simulink model "zero_to_hero_sect11_pid"  (R2023a)
settings: Solver=VariableStepAuto  StartTime=0.0  StopTime=simtime  MaxStep=0.01  RelTol=1e-3
values from neighbouring files (symbols this model uses):
  b = 50    [zero_to_hero_sect10_script.m]    (also in zero_to_hero_sect1to5_script.m = 0.1; zero_to_hero_sect7to8_script.m = 10)
undefined symbols (not defined in the file or in its folder): J_Mo, K_m, L, R, target_angular_vel
libraries: slpidlib x1
settings Model: Creator=fycce  LastModifiedBy=fycce
settings DataIOCC: SaveOutput=off  SaveTime=off  ReturnWorkspaceOutputs=off

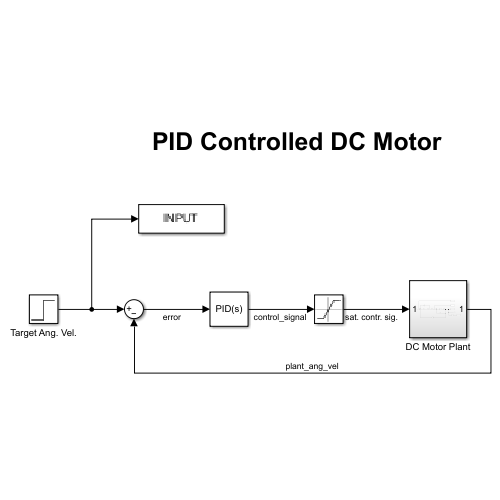
[thumbnail: Simulink's stored preview of the top-level diagram]
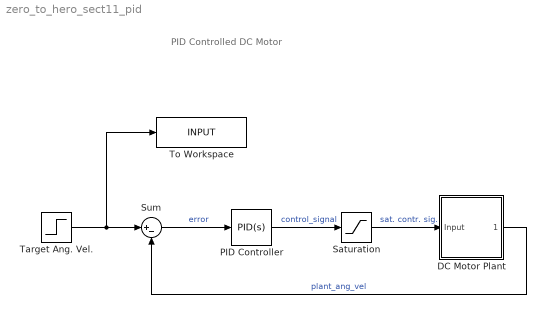
== system zero_to_hero_sect11_pid ==
  note: PID Controlled DC Motor
  DC Motor Plant : Subsystem
  PID Controller : slpidlib/PID Controller  Controller=PID  Form=Parallel  TimeDomain=Continuous-time  UseExternalTs=off  SampleTime=-1  IntegratorMethod=Forward Euler  FilterMethod=Forward Euler  ControllerParametersSource=internal  P=17.19  I=204.8  UseKiTs=off  D=0.2523  N=1422  UseFilter=on  TunerSelectOption=Transfer Function Based (PID Tuner App)  InitialConditionSource=internal  InitialConditionForIntegrator=0  InitialConditionForFilter=0  DifferentiatorICPrevScaledInput=0  ExternalReset=none  TrackingMode=off  Kt=1  LimitOutput=off  SatLimitsSource=internal  UpperSaturationLimit=inf  LowerSaturationLimit=-inf  LinearizeAsGain=on  AntiWindupMode=none  Kb=1  LimitIntegrator=off  UpperIntegratorSaturationLimit=inf  LowerIntegratorSaturationLimit=-inf  POutMin=[]  POutMax=[]  IOutMin=[]  IOutMax=[]  DOutMin=[]  DOutMax=[]  NOutMin=[]  NOutMax=[]  SumOutMin=[]  SumOutMax=[]  SaturationOutMin=[]  SaturationOutMax=[]  PParamMin=[]  PParamMax=[]  IParamMin=[]  IParamMax=[]  DParamMin=[]  DParamMax=[]  NParamMin=[]  NParamMax=[]  KbParamMin=[]  KbParamMax=[]  KtParamMin=[]  KtParamMax=[]  KbOutMin=[]  KbOutMax=[]  KtOutMin=[]  KtOutMax=[]  IntegratorOutMin=[]  IntegratorOutMax=[]  FilterOutMin=[]  FilterOutMax=[]  SumI1OutMin=[]  SumI1OutMax=[]  SumI2OutMin=[]  SumI2OutMax=[]  SumI3OutMin=[]  SumI3OutMax=[]  SumI4OutMin=[]  SumI4OutMax=[]  SumDOutMin=[]  SumDOutMax=[]  DifferentiatorOutMin=[]  DifferentiatorOutMax=[]  FilterDiffOutCoefMin=[]  FilterDiffOutCoefMax=[]  ReciprocalOutMin=[]  ReciprocalOutMax=[]  SumDenOutMin=[]  SumDenOutMax=[]  SumNumOutMin=[]  SumNumOutMax=[]  DivideOutMin=[]  DivideOutMax=[]  UdiffTsProdOutMin=[]  UdiffTsProdOutMax=[]  NTsProdOutMin=[]  NTsProdOutMax=[]  UintegralTsProdOutMin=[]  UintegralTsProdOutMax=[]  UngainTsProdOutMin=[]  UngainTsProdOutMax=[]  ClampingZeroOutDataTypeStr=Inherit: Inherit via back propagation  ClampingZeroOutMin=[]  ClampingZeroOutMax=[]  FilterDenConstantOutDataTypeStr=Inherit: Inherit via back propagation  FilterDenConstantOutMin=[]  FilterDenConstantOutMax=[]  PCopyOutDataTypeStr=Inherit: Inherit via back propagation  PCopyOutMin=[]  PCopyOutMax=[]  NCopyOutDataTypeStr=Inherit: Inherit via back propagation  NCopyOutMin=[]  NCopyOutMax=[]  IntegratorContinuousStateAttributes=''  IntegratorStateMustResolveToSignalObject=off  IntegratorRTWStateStorageClass=Auto  FilterContinuousStateAttributes=''  FilterStateMustResolveToSignalObject=off  FilterRTWStateStorageClass=Auto  ParallelPVariant=InternalParameters  IdealPVariant=Disabled  IVariant=InternalParameters  DVariant=InternalParameters  IntegratorVariant=Continuous  SatVariant=Disabled  AWVariant=Passthrough  PCopyVariant=Disabled  TRVariant=Disabled  FdbkBlocksVariant=Forward  IdealPFdbkVariant=Disabled  SatFdbkVariant=Disabled  DerivativeFilterVariant=ContFilter  NVariant=InternalParameters  NCopyVariant=Disabled  FilterICVariant=InternalICsFilter  IntegratorICVariant=InternalICs  ExternalResetVariant=Disabled  TRSumVariant=Passthrough  SumFdbkVariant=Disabled  SumVariant=Sum_PID  TsampFilterVariant=InternalTs  TsampNgainVariant=Passthrough  TsampIntegralVariant=Disabled_SignalSpec  ExternalSaturationOutDataTypeStr=Inherit: Same as second input
  Saturation : Saturate  UpperLimit=24  LowerLimit=-24
  Sum : Sum  Inputs=|+-
  Target Ang. Vel. : Step  Time=0  After=target_angular_vel  SampleTime=0
  To Workspace : ToWorkspace  VariableName=INPUT  SaveFormat=Timeseries  SampleTime=-1
  wires:
  DC Motor Plant/1(Output) -> Sum/2  "plant_ang_vel"
  Sum/1 -> PID Controller/1  "error"
  Target Ang. Vel./1 -> To Workspace/1, Sum/1
  PID Controller/1 -> Saturation/1  "control_signal"
  Saturation/1 -> DC Motor Plant/1(Input)  "sat. contr. sig."

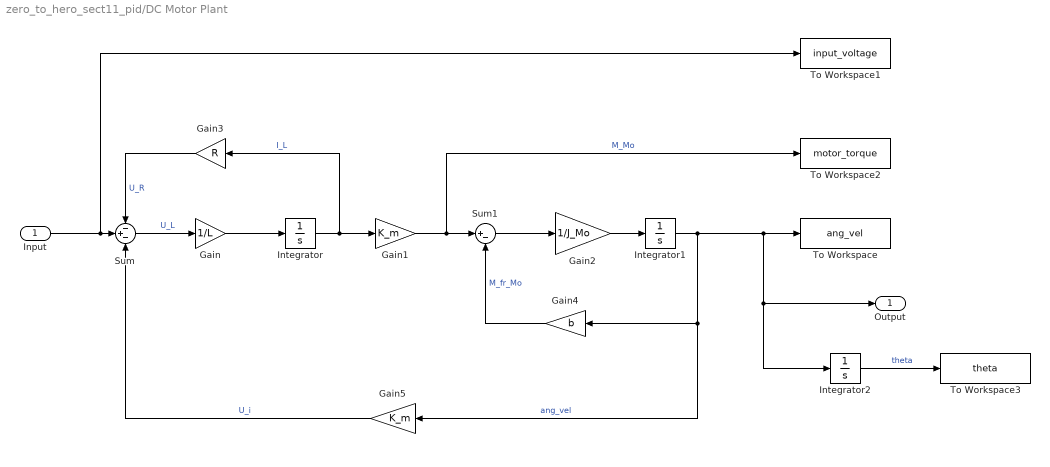
== system zero_to_hero_sect11_pid/DC Motor Plant ==
  Input : Inport
  Gain : Gain  Gain=1/L
  Gain1 : Gain  Gain=K_m
  Gain2 : Gain  Gain=1/J_Mo
  Gain3 : Gain  Gain=R
  Gain4 : Gain  Gain=b
  Gain5 : Gain  Gain=K_m
  Integrator : Integrator
  Integrator1 : Integrator
  Integrator2 : Integrator
  Sum : Sum  Inputs=-+-
  Sum1 : Sum  Inputs=|+-
  To Workspace : ToWorkspace  VariableName=ang_vel  SaveFormat=Timeseries  SampleTime=-1
  To Workspace1 : ToWorkspace  VariableName=input_voltage  SaveFormat=Timeseries  SampleTime=-1
  To Workspace2 : ToWorkspace  VariableName=motor_torque  SaveFormat=Timeseries  SampleTime=-1
  To Workspace3 : ToWorkspace  VariableName=theta  SaveFormat=Timeseries  SampleTime=-1
  Output : Outport
  wires:
  Integrator2/1 -> To Workspace3/1  "theta"
  Integrator1/1 -> Gain4/1, Gain5/1, To Workspace/1, Output/1, Integrator2/1  "ang_vel"
  Sum/1 -> Gain/1  "U_L"
  Sum1/1 -> Gain2/1
  Gain1/1 -> To Workspace2/1, Sum1/1  "M_Mo"
  Gain4/1 -> Sum1/2  "M_fr_Mo"
  Gain/1 -> Integrator/1
  Input/1 -> To Workspace1/1, Sum/2
  Gain3/1 -> Sum/1  "U_R"
  Gain2/1 -> Integrator1/1
  Integrator/1 -> Gain3/1, Gain1/1  "I_L"
  Gain5/1 -> Sum/3  "U_i"
